simulink library "BrakePressure"  (R2024a)
settings: Solver=VariableStepAuto  StartTime=0.0  StopTime=10.0  RelTol=1e-3
undefined symbols (not defined in the file or in its folder): raptor_xcp_function, StateSignal
libraries: Raptor_lib x5, Utilities x4, simulink x4
settings Model: Creator=serga  LastModifiedBy=serga

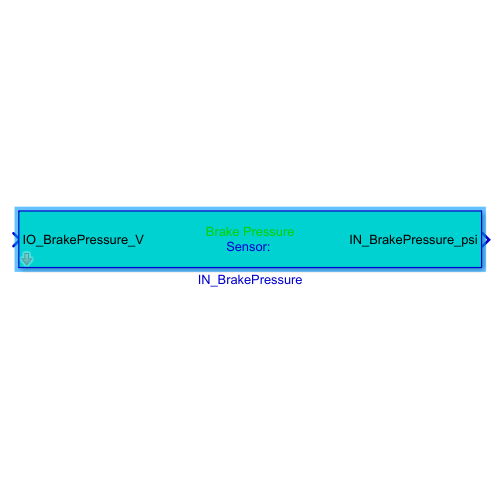
[thumbnail: Simulink's stored preview of the top-level diagram]
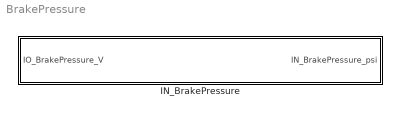
== system BrakePressure ==
  IN_BrakePressure : Subsystem  mask{pos=''}
      mask prompts: pos "Position"
      mask Display:
      | color('green')
      | disp('Brake Pressure\n');
      | color('blue')
      | disp(['\nSensor: ' pos]);
      | color('black')
      | port_label('input', 1, ['IO_BrakePressure' pos '_V']);
      | port_label('output', 1, ['IN_BrakePressure' pos '_psi']);

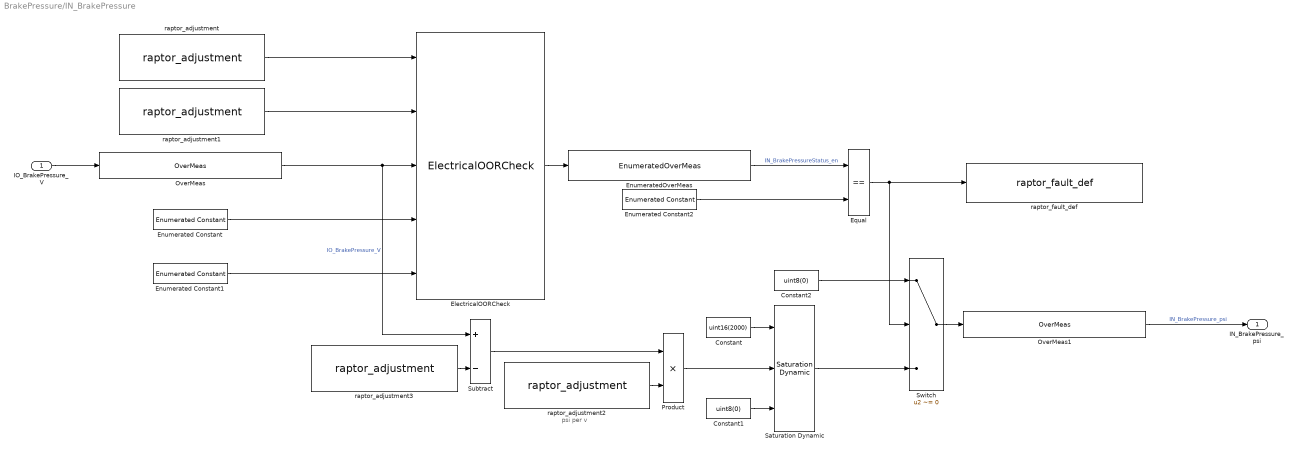
== system BrakePressure/IN_BrakePressure ==
  note: psi per v
  IO_BrakePressure_V : Inport
  Constant : Constant  Value=uint16(2000)
  Constant1 : Constant  Value=uint8(0)
  Constant2 : Constant  Value=uint8(0)
  ElectricalOORCheck : Utilities/ElectricalOORCheck
  Enumerated Constant : simulink/Sources/Enumerated Constant  OutDataTypeStr=Enum: StateSignal  Value=StateSignal.Normal  SampleTime=inf
  Enumerated Constant1 : simulink/Sources/Enumerated Constant  OutDataTypeStr=Enum: StateSignal  Value=StateSignal.Fault  SampleTime=inf
  Enumerated Constant2 : simulink/Sources/Enumerated Constant  OutDataTypeStr=Enum: StateSignal  Value=StateSignal.Fault  SampleTime=inf
  EnumeratedOverMeas : Utilities/EnumeratedOverMeas  sigName=['IN_BrakePressure' pos 'Status_en']  enumName='StateSignal'
  Equal : RelationalOperator  Operator===  OutDataTypeStr=boolean  RndMeth=Simplest  InputSameDT=off
  OverMeas : Utilities/OverMeas  sigName=['IO_BrakePressure' pos '_V']  minimum=0  maximum=5
  OverMeas1 : Utilities/OverMeas  sigName=['IN_BrakePressure' pos '_psi']  minimum=0  maximum=2500
  Product : Product
  Saturation Dynamic : simulink/Discontinuities/Saturation Dynamic  OutMin=[]  OutMax=[]  OutDataTypeStr=Inherit: Same as second input  OutDataType=fixdt(1, 16)  OutScaling=2^-10  DoSatur=off
  Subtract : Sum  Inputs=+-
  Switch : Switch  Criteria=u2 ~= 0  SaturateOnIntegerOverflow=off  InputSameDT=off
  raptor_adjustment : Raptor_lib/Data Storage/raptor_adjustment  paramName=['IN_BrakePressure' pos 'HighThresh_V']  nameSource=Parameter  initValue=4.5  dataType=single  storage=Calibration  calDispType=Number  calEnum={'False', 'True'}  calGain=1.0  calOffset=0.0  calMax=5  calMin=0  calFormat='-1'  calUnit=''  calHelp=''  calAccess=1  calFunction=raptor_xcp_function(gcb)  calDispHeaders=off  calColHeaders={'Col1' 'Col2' 'Col3'}  calRowHeaders={'Row1' 'Row2' 'Row3'}
      settings: SourceProductName=Raptor
  raptor_adjustment1 : Raptor_lib/Data Storage/raptor_adjustment  paramName=['IN_BrakePressure' pos 'LowThresh_V']  nameSource=Parameter  initValue=0.4  dataType=single  storage=Calibration  calDispType=Number  calEnum={'False', 'True'}  calGain=1.0  calOffset=0.0  calMax=5  calMin=0  calFormat='-1'  calUnit=''  calHelp=''  calAccess=1  calFunction=raptor_xcp_function(gcb)  calDispHeaders=off  calColHeaders={'Col1' 'Col2' 'Col3'}  calRowHeaders={'Row1' 'Row2' 'Row3'}
      settings: SourceProductName=Raptor
  raptor_adjustment2 : Raptor_lib/Data Storage/raptor_adjustment  paramName=['IN_BrakePressure' pos 'Scale_na']  nameSource=Parameter  initValue=500  dataType=single  storage=Calibration  calDispType=Number  calEnum={'False', 'True'}  calGain=1.0  calOffset=0.0  calMax=inf  calMin=-inf  calFormat='-1'  calUnit=''  calHelp=''  calAccess=1  calFunction=raptor_xcp_function(gcb)  calDispHeaders=off  calColHeaders={'Col1' 'Col2' 'Col3'}  calRowHeaders={'Row1' 'Row2' 'Row3'}
      settings: SourceProductName=Raptor
  raptor_adjustment3 : Raptor_lib/Data Storage/raptor_adjustment  paramName=['IN_BrakePressure' pos 'Zero_V']  nameSource=Parameter  initValue=0.49  dataType=single  storage=Calibration  calDispType=Number  calEnum={'False', 'True'}  calGain=1.0  calOffset=0.0  calMax=5  calMin=0  calFormat='-1'  calUnit=''  calHelp=''  calAccess=1  calFunction=raptor_xcp_function(gcb)  calDispHeaders=off  calColHeaders={'Col1' 'Col2' 'Col3'}  calRowHeaders={'Row1' 'Row2' 'Row3'}
      settings: SourceProductName=Raptor
  raptor_fault_def : Raptor_lib/Faults/raptor_fault_def  faultName=['IN_BrakePressure' pos 'Fault']  persist=off  sticky=off  emisRelated=off  singleTrip=off  clearMethod=Standard  xLimit=25  yLimit=50  calEnable=on  addDisable=off  calAccess=1  calFunction='System | FaultManager'
      settings: SourceProductName=Raptor
  IN_BrakePressure_psi : Outport
  wires:
  IO_BrakePressure_V/1 -> OverMeas/1
  OverMeas/1 -> Subtract/1, ElectricalOORCheck/3  "IO_BrakePressure_V"
  raptor_adjustment/1 -> ElectricalOORCheck/1
  raptor_adjustment1/1 -> ElectricalOORCheck/2
  Enumerated Constant/1 -> ElectricalOORCheck/4
  Enumerated Constant1/1 -> ElectricalOORCheck/5
  ElectricalOORCheck/1 -> EnumeratedOverMeas/1
  Enumerated Constant2/1 -> Equal/2
  Equal/1 -> Switch/2, raptor_fault_def/1
  EnumeratedOverMeas/1 -> Equal/1  "IN_BrakePressureStatus_en"
  raptor_adjustment2/1 -> Product/2
  raptor_adjustment3/1 -> Subtract/2
  Subtract/1 -> Product/1
  Product/1 -> Saturation Dynamic/2
  Saturation Dynamic/1 -> Switch/3
  Constant/1 -> Saturation Dynamic/1
  Constant1/1 -> Saturation Dynamic/3
  Constant2/1 -> Switch/1
  OverMeas1/1 -> IN_BrakePressure_psi/1  "IN_BrakePressure_psi"
  Switch/1 -> OverMeas1/1
